simulink model "Phase_Estimation_tunable_2nd"  (Simulink 8.7)
settings: Solver=ode3  StartTime=0.0  StopTime=t(end)  FixedStep=1/60  RelTol=1e-3
values from neighbouring files (symbols this model uses):
  Data = [0:1/60:400]'    [Adaptive_notch_filter.m]    (also in Evolutionary_Strategy_ANF_mutation.m)
  gamma_d = 0.0324    [Adaptive_notch_filter.m]    (also in Evolutionary_Strategy_ANF_mutation.m = mean(Gamma_d))
  gamma_omg = 2.0893*10^(-10)    (= 2.0893e-10)    [Adaptive_notch_filter.m]    (also in Evolutionary_Strategy_ANF_mutation.m = mean(Gamma_omg))
  x_initial = [0 0 0 0 0 0 0 0 0 0 0 2*pi/24]    [Adaptive_notch_filter.m]    (also in Evolutionary_Strategy_ANF_mutation.m = [0 0 0 0 0 0 0 2*pi/24])
  zeta = 0.0599    [Adaptive_notch_filter.m]    (also in Evolutionary_Strategy_ANF_mutation.m = mean(Zeta))
settings Model: Creator=wangf7  LastModifiedBy=Jiawei Yin
settings OptimizationCC: ExpressionDepthLimit=2147483647
settings DebuggingCC: SolverPrmCheckMsg=warning  StateNameClashWarn=warning
settings ConfigurationSet: Description=SimMechanics 2G

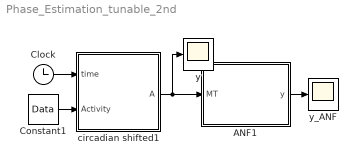
== system Phase_Estimation_tunable_2nd ==
  ANF1 : Subsystem
  Clock : Clock
  Constant1 : Constant  Value=Data
  circadian shifted1 : MATLAB Function  TreatAsAtomicUnit=on
  y : Scope
  y_ANF : Scope
  wires:
  circadian shifted1/1(A) -> y/1, ANF1/1(MT)
  Constant1/1 -> circadian shifted1/2(Activity)
  Clock/1 -> circadian shifted1/1(time)
  ANF1/1(y) -> y_ANF/1

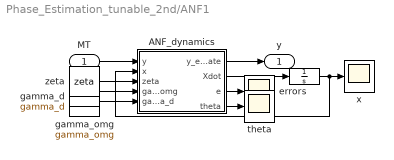
== system Phase_Estimation_tunable_2nd/ANF1 ==
  MT : Inport
  ANF_dynamics : MATLAB Function  TreatAsAtomicUnit=on
  error : Scope
  gamma_d : Constant  Value=gamma_d
  gamma_omg : Constant  Value=gamma_omg
  s : Integrator  InitialCondition=x_initial
  theta : Scope
  x : Scope
  zeta : Constant  Value=zeta
  y : Outport
  wires:
  MT/1 -> ANF_dynamics/1(y)
  s/1 -> ANF_dynamics/2(x), x/1
  ANF_dynamics/2(Xdot) -> s/1
  ANF_dynamics/1(y_estimate) -> y/1
  ANF_dynamics/3(e) -> error/1
  ANF_dynamics/4(theta) -> theta/1
  zeta/1 -> ANF_dynamics/3(zeta)
  gamma_omg/1 -> ANF_dynamics/4(gamma_omg)
  gamma_d/1 -> ANF_dynamics/5(gamma_d)

== matlab function circadian shifted1 ==
  data: time input double; Activity input double; A output double
function A = fcn(time,Activity)
%#eml
A=interp1q(Activity(:,1),Activity(:,2),time);

== matlab function ANF1/ANF_dynamics ==
  data: y_estimate output double; y input double; x input double; zeta input double; Xdot output double; e output double; theta output double; gamma_omg input double; gamma_d input double
function [y_estimate,Xdot,e,theta] = fcn(y,x,zeta,gamma_omg,gamma_d)

x1 = x(1);%1st harmonic
x2 = x(2);%1st harmonic dot
x3 = x(3);%2nd harmonic
x4 = x(4);%2nd harmonic dot
dc = x(5);%dc
omg = x(6);%omega

y_estimate = dc + 2*zeta/omg*x2  + zeta/omg*x4;
e = y - y_estimate;
if isnan(y)
    e=0;
end

Xdot = zeros(6,1);

Xdot(1,1) = x2;
Xdot(2,1) = omg^2*(e-x1);
Xdot(3,1) = x4;
Xdot(4,1) = (2*omg)^2*(e-x3);
Xdot(5,1) = gamma_d*e;
Xdot(6,1) = gamma_omg*(-x1*omg^2)*e;
%y_estimate = dc + 2*zeta/omg*x2;
theta=mod(atan2(x(2),-x(6)*x(1)),2*pi);
